simulink model "Simulink_TEP"  (R2024a)
settings: Solver=FixedStepAuto  StartTime=0.0  StopTime=5  FixedStep=1/3600  RelTol=1e-3
model workspace (MAT data in the model file):
  AD : Simulink.Parameter (value not decoded)
  AG : Simulink.Parameter (value not decoded)
  AH : Simulink.Parameter (value not decoded)
  AV : Simulink.Parameter (value not decoded)
  AVP : Simulink.Parameter (value not decoded)
  BCHL : Simulink.Parameter (value not decoded)
  BCHV : Simulink.Parameter (value not decoded)
  BD : Simulink.Parameter (value not decoded)
  BG : Simulink.Parameter (value not decoded)
  BH : Simulink.Parameter (value not decoded)
  BVP : Simulink.Parameter (value not decoded)
  CD : Simulink.Parameter (value not decoded)
  CG : Simulink.Parameter (value not decoded)
  CH : Simulink.Parameter (value not decoded)
  CVP : Simulink.Parameter (value not decoded)
  XMW : Simulink.Parameter (value not decoded)
symbols that are objects in the model workspace (value not decoded): AD, AG, AH, AV, AVP, BD, BG, BH, BVP, CD, CG, CH, CVP, XMW
undefined symbols (not defined in the file or in its folder): magnitude, SETPT, XMEAS, XMV
libraries: mylib x165, dspindex x17
(part 9 of 10)

== system Simulink_TEP/Subsystem/Braatz/ 9/CONTROL 16 ==
  XMEAS(18) : Inport
  SETPT(16) : Inport  Port=2
  Constant1 : Constant  Value=GAIN16
  Constant2 : Constant  Value=TAUI16
  Constant3 : Constant  Value=HIGH16
  Constant5 : Constant  Value=SI16
  Constant6 : Constant  Value=HIGH9
  PI Control Setpoint : mylib/Braatz Control/PI Control Setpoint  SystemSampleTime=-1  VariantActivationTime=update diagram  AllowFlexibleInterface=on  Latency=0  AutoFrameSizeCalculation=off
  Sampling interval : mylib/Braatz Control/Sampling interval  SystemSampleTime=-1  VariantActivationTime=update diagram  AllowFlexibleInterface=on  Latency=0  AutoFrameSizeCalculation=off
  Unit Delay : UnitDelay  InitialCondition=SETPT9  SampleTime=-1  HasFrameUpgradeWarning=on
  Unit Delay1 : UnitDelay  SampleTime=-1  HasFrameUpgradeWarning=on
  SETPT(9) : Outport  VectorParamsAs1DForOutWhenUnconnected=off
  wires:
  Sampling interval/1 -> PI Control Setpoint/Action
  SETPT(16)/1 -> PI Control Setpoint/1
  XMEAS(18)/1 -> PI Control Setpoint/2
  PI Control Setpoint/1 -> SETPT(9)/1, Unit Delay/1
  Constant2/1 -> PI Control Setpoint/8
  Constant5/1 -> PI Control Setpoint/7, Sampling interval/1
  Constant1/1 -> PI Control Setpoint/6
  Constant3/1 -> PI Control Setpoint/3
  Unit Delay/1 -> PI Control Setpoint/4
  Constant6/1 -> PI Control Setpoint/5
  PI Control Setpoint/2 -> Unit Delay1/1
  Unit Delay1/1 -> PI Control Setpoint/9

== system Simulink_TEP/Subsystem/Braatz/ 9/CONTROL 20 ==
  XMEAS(38) : Inport
  Constant : Constant  Value=SETPT20
  Constant1 : Constant  Value=GAIN20
  Constant2 : Constant  Value=TAUI20
  Constant3 : Constant  Value=HIGH20
  Constant5 : Constant  Value=SI20
  Constant6 : Constant  Value=HIGH16
  PI Control Setpoint : mylib/Braatz Control/PI Control Setpoint  SystemSampleTime=-1  VariantActivationTime=update diagram  AllowFlexibleInterface=on  Latency=0  AutoFrameSizeCalculation=off
  Sampling interval : mylib/Braatz Control/Sampling interval  SystemSampleTime=-1  VariantActivationTime=update diagram  AllowFlexibleInterface=on  Latency=0  AutoFrameSizeCalculation=off
  Unit Delay : UnitDelay  InitialCondition=SETPT16  SampleTime=-1  HasFrameUpgradeWarning=on
  Unit Delay1 : UnitDelay  SampleTime=-1  HasFrameUpgradeWarning=on
  SETPT(16) : Outport  VectorParamsAs1DForOutWhenUnconnected=off
  wires:
  Sampling interval/1 -> PI Control Setpoint/Action
  Constant/1 -> PI Control Setpoint/1
  XMEAS(38)/1 -> PI Control Setpoint/2
  PI Control Setpoint/1 -> SETPT(16)/1, Unit Delay/1
  Constant2/1 -> PI Control Setpoint/8
  Constant5/1 -> PI Control Setpoint/7, Sampling interval/1
  Constant1/1 -> PI Control Setpoint/6
  Constant3/1 -> PI Control Setpoint/3
  Unit Delay/1 -> PI Control Setpoint/4
  Constant6/1 -> PI Control Setpoint/5
  PI Control Setpoint/2 -> Unit Delay1/1
  Unit Delay1/1 -> PI Control Setpoint/9

== system Simulink_TEP/Subsystem/Braatz/ 9/CONTROL 9 ==
  XMEAS(19) : Inport
  SETPT(9) : Inport  Port=2
  Constant1 : Constant  Value=GAIN9
  Constant2 : Constant  Value=HIGH9
  Constant3 : Constant  Value=SI9
  P Control : mylib/Braatz Control/P Control  SystemSampleTime=-1  VariantActivationTime=update diagram  AllowFlexibleInterface=on  Latency=0  AutoFrameSizeCalculation=off
  Sampling interval : mylib/Braatz Control/Sampling interval  SystemSampleTime=-1  VariantActivationTime=update diagram  AllowFlexibleInterface=on  Latency=0  AutoFrameSizeCalculation=off
  Unit Delay : UnitDelay  InitialCondition=XMV9_0  SampleTime=-1  HasFrameUpgradeWarning=on
  Unit Delay1 : UnitDelay  SampleTime=-1  HasFrameUpgradeWarning=on
  XMV(9) : Outport  VectorParamsAs1DForOutWhenUnconnected=off
  wires:
  Constant2/1 -> P Control/5
  Constant1/1 -> P Control/3
  SETPT(9)/1 -> P Control/1
  Unit Delay/1 -> P Control/2
  XMEAS(19)/1 -> P Control/4
  P Control/1 -> XMV(9)/1, Unit Delay/1
  Sampling interval/1 -> P Control/Action
  Constant3/1 -> Sampling interval/1
  P Control/2 -> Unit Delay1/1
  Unit Delay1/1 -> P Control/6

== system Simulink_TEP/Disturbances/Subsystem1/Subsystem2/If Action Subsystem/Subsystem ==
  Bus Creator : BusCreator  Inputs=5
  HSPAN(2) : Constant  Value=0.7
  HZERO(2) : Constant
  SPSPAN(2) : Constant  Value=0
  SSPAN(2) : Constant  Value=0.003
  SZERO(2) : Constant  Value=0.005
  Out1 : Outport  VectorParamsAs1DForOutWhenUnconnected=off
  wires:
  SSPAN(2)/1 -> Bus Creator/3  "SSPAN"
  HSPAN(2)/1 -> Bus Creator/1  "HSPAN"
  Bus Creator/1 -> Out1/1
  SPSPAN(2)/1 -> Bus Creator/5  "SPSPAN"
  HZERO(2)/1 -> Bus Creator/2  "HZERO"
  SZERO(2)/1 -> Bus Creator/4  "SZERO"

== system Simulink_TEP/Disturbances/Subsystem1/Subsystem2/If Action Subsystem1/Subsystem1 ==
  BDIST(2) : Constant  Value=0
  Bus Creator : BusCreator  Inputs=6
  CDIST(2) : Constant  Value=0
  DDIST(2) : Constant  Value=0
  SZERO(2) : Constant  Value=0.005
  TENXT(2) : Constant  Value=0.1
  TLAST(2) : Constant  Value=0
  DIST : Outport  VectorParamsAs1DForOutWhenUnconnected=off
  wires:
  Bus Creator/1 -> DIST/1
  TENXT(2)/1 -> Bus Creator/5  "TNEXT"
  SZERO(2)/1 -> Bus Creator/1  "ADIST"
  TLAST(2)/1 -> Bus Creator/6  "TLAST"
  DDIST(2)/1 -> Bus Creator/4  "DDIST"
  BDIST(2)/1 -> Bus Creator/2  "BDIST"
  CDIST(2)/1 -> Bus Creator/3  "CDIST"

== system Simulink_TEP/Disturbances/Subsystem10/Subsystem3/If Action Subsystem/Subsystem2 ==
  Bus Creator : BusCreator  Inputs=5
  HSPAN(10) : Constant  Value=1.5
  HZERO(10) : Constant  Value=2
  SPSPAN(10) : Constant  Value=0
  SSPAN(10) : Constant  Value=0
  SZERO(10) : Constant  Value=0
  Out1 : Outport  VectorParamsAs1DForOutWhenUnconnected=off
  wires:
  SSPAN(10)/1 -> Bus Creator/3  "SSPAN"
  HSPAN(10)/1 -> Bus Creator/1  "HSPAN"
  Bus Creator/1 -> Out1/1
  SPSPAN(10)/1 -> Bus Creator/5  "SPSPAN"
  HZERO(10)/1 -> Bus Creator/2  "HZERO"
  SZERO(10)/1 -> Bus Creator/4  "SZERO"

== system Simulink_TEP/Disturbances/Subsystem10/Subsystem3/If Action Subsystem1/Subsystem1 ==
  BDIST(10) : Constant  Value=0
  Bus Creator : BusCreator  Inputs=6
  CDIST(10) : Constant  Value=0
  DDIST(10) : Constant  Value=0
  SZERO(10) : Constant  Value=0
  TENXT(10) : Constant  Value=0.1
  TLAST(10) : Constant  Value=0
  DIST : Outport  VectorParamsAs1DForOutWhenUnconnected=off
  wires:
  Bus Creator/1 -> DIST/1
  TENXT(10)/1 -> Bus Creator/5  "TNEXT"
  SZERO(10)/1 -> Bus Creator/1  "ADIST"
  TLAST(10)/1 -> Bus Creator/6  "TLAST"
  DDIST(10)/1 -> Bus Creator/4  "DDIST"
  BDIST(10)/1 -> Bus Creator/2  "BDIST"
  CDIST(10)/1 -> Bus Creator/3  "CDIST"

== system Simulink_TEP/Disturbances/Subsystem11/Subsystem3/If Action Subsystem/Subsystem2 ==
  Bus Creator : BusCreator  Inputs=5
  HSPAN(11) : Constant  Value=2
  HZERO(11) : Constant  Value=3
  SPSPAN(11) : Constant  Value=0
  SSPAN(11) : Constant  Value=0
  SZERO(11) : Constant  Value=0
  Out1 : Outport  VectorParamsAs1DForOutWhenUnconnected=off
  wires:
  SSPAN(11)/1 -> Bus Creator/3  "SSPAN"
  HSPAN(11)/1 -> Bus Creator/1  "HSPAN"
  Bus Creator/1 -> Out1/1
  SPSPAN(11)/1 -> Bus Creator/5  "SPSPAN"
  HZERO(11)/1 -> Bus Creator/2  "HZERO"
  SZERO(11)/1 -> Bus Creator/4  "SZERO"

== system Simulink_TEP/Disturbances/Subsystem11/Subsystem3/If Action Subsystem1/Subsystem1 ==
  BDIST(11) : Constant  Value=0
  Bus Creator : BusCreator  Inputs=6
  CDIST(11) : Constant  Value=0
  DDIST(11) : Constant  Value=0
  SZERO(11) : Constant  Value=0
  TENXT(11) : Constant  Value=0.1
  TLAST(11) : Constant  Value=0
  DIST : Outport  VectorParamsAs1DForOutWhenUnconnected=off
  wires:
  Bus Creator/1 -> DIST/1
  TENXT(11)/1 -> Bus Creator/5  "TNEXT"
  SZERO(11)/1 -> Bus Creator/1  "ADIST"
  TLAST(11)/1 -> Bus Creator/6  "TLAST"
  DDIST(11)/1 -> Bus Creator/4  "DDIST"
  BDIST(11)/1 -> Bus Creator/2  "BDIST"
  CDIST(11)/1 -> Bus Creator/3  "CDIST"

== system Simulink_TEP/Disturbances/Subsystem12/Subsystem3/If Action Subsystem/Subsystem2 ==
  Bus Creator : BusCreator  Inputs=5
  HSPAN(12) : Constant  Value=1.5
  HZERO(12) : Constant  Value=2
  SPSPAN(12) : Constant  Value=0
  SSPAN(12) : Constant  Value=0
  SZERO(12) : Constant  Value=0
  Out1 : Outport  VectorParamsAs1DForOutWhenUnconnected=off
  wires:
  SSPAN(12)/1 -> Bus Creator/3  "SSPAN"
  HSPAN(12)/1 -> Bus Creator/1  "HSPAN"
  Bus Creator/1 -> Out1/1
  SPSPAN(12)/1 -> Bus Creator/5  "SPSPAN"
  HZERO(12)/1 -> Bus Creator/2  "HZERO"
  SZERO(12)/1 -> Bus Creator/4  "SZERO"

== system Simulink_TEP/Disturbances/Subsystem12/Subsystem3/If Action Subsystem1/Subsystem1 ==
  BDIST(12) : Constant  Value=0
  Bus Creator : BusCreator  Inputs=6
  CDIST(12) : Constant  Value=0
  DDIST(12) : Constant  Value=0
  SZERO(12) : Constant  Value=0
  TENXT(12) : Constant  Value=0.1
  TLAST(12) : Constant  Value=0
  DIST : Outport  VectorParamsAs1DForOutWhenUnconnected=off
  wires:
  Bus Creator/1 -> DIST/1
  TENXT(12)/1 -> Bus Creator/5  "TNEXT"
  SZERO(12)/1 -> Bus Creator/1  "ADIST"
  TLAST(12)/1 -> Bus Creator/6  "TLAST"
  DDIST(12)/1 -> Bus Creator/4  "DDIST"
  BDIST(12)/1 -> Bus Creator/2  "BDIST"
  CDIST(12)/1 -> Bus Creator/3  "CDIST"

== system Simulink_TEP/Disturbances/Subsystem2/Subsystem/If Action Subsystem/Subsystem ==
  Bus Creator : BusCreator  Inputs=5
  HSPAN(1) : Constant  Value=0.2
  HZERO(1) : Constant  Value=0.5
  SPSPAN(1) : Constant  Value=0
  SSPAN(1) : Constant  Value=0.03
  SZERO(1) : Constant  Value=0.485
  Out1 : Outport  VectorParamsAs1DForOutWhenUnconnected=off
  wires:
  SSPAN(1)/1 -> Bus Creator/3  "SSPAN"
  HSPAN(1)/1 -> Bus Creator/1  "HSPAN"
  Bus Creator/1 -> Out1/1
  SPSPAN(1)/1 -> Bus Creator/5  "SPSPAN"
  HZERO(1)/1 -> Bus Creator/2  "HZERO"
  SZERO(1)/1 -> Bus Creator/4  "SZERO"

== system Simulink_TEP/Disturbances/Subsystem2/Subsystem/If Action Subsystem1/Subsystem1 ==
  BDIST(1) : Constant  Value=0
  Bus Creator : BusCreator  Inputs=6
  CDIST(1) : Constant  Value=0
  DDIST(1) : Constant  Value=0
  SZERO(1) : Constant  Value=0.485
  TENXT(1) : Constant  Value=0.1
  TLAST(1) : Constant  Value=0
  DIST : Outport  VectorParamsAs1DForOutWhenUnconnected=off
  wires:
  Bus Creator/1 -> DIST/1
  TENXT(1)/1 -> Bus Creator/5  "TNEXT"
  SZERO(1)/1 -> Bus Creator/1  "ADIST"
  TLAST(1)/1 -> Bus Creator/6  "TLAST"
  DDIST(1)/1 -> Bus Creator/4  "DDIST"
  BDIST(1)/1 -> Bus Creator/2  "BDIST"
  CDIST(1)/1 -> Bus Creator/3  "CDIST"

== system Simulink_TEP/Disturbances/Subsystem3/Subsystem2/If Action Subsystem/Subsystem ==
  Bus Creator : BusCreator  Inputs=5
  HSPAN(3) : Constant  Value=0.25
  HZERO(3) : Constant  Value=0.5
  SPSPAN(3) : Constant  Value=0
  SSPAN(3) : Constant  Value=10
  SZERO(3) : Constant  Value=45
  Out1 : Outport  VectorParamsAs1DForOutWhenUnconnected=off
  wires:
  SSPAN(3)/1 -> Bus Creator/3  "SSPAN"
  HSPAN(3)/1 -> Bus Creator/1  "HSPAN"
  Bus Creator/1 -> Out1/1
  SPSPAN(3)/1 -> Bus Creator/5  "SPSPAN"
  HZERO(3)/1 -> Bus Creator/2  "HZERO"
  SZERO(3)/1 -> Bus Creator/4  "SZERO"

== system Simulink_TEP/Disturbances/Subsystem3/Subsystem2/If Action Subsystem1/Subsystem1 ==
  BDIST(3) : Constant  Value=0
  Bus Creator : BusCreator  Inputs=6
  CDIST(3) : Constant  Value=0
  DDIST(3) : Constant  Value=0
  SZERO(3) : Constant  Value=45
  TENXT(3) : Constant  Value=0.1
  TLAST(3) : Constant  Value=0
  DIST : Outport  VectorParamsAs1DForOutWhenUnconnected=off
  wires:
  Bus Creator/1 -> DIST/1
  TENXT(3)/1 -> Bus Creator/5  "TNEXT"
  SZERO(3)/1 -> Bus Creator/1  "ADIST"
  TLAST(3)/1 -> Bus Creator/6  "TLAST"
  DDIST(3)/1 -> Bus Creator/4  "DDIST"
  BDIST(3)/1 -> Bus Creator/2  "BDIST"
  CDIST(3)/1 -> Bus Creator/3  "CDIST"

== system Simulink_TEP/Disturbances/Subsystem4/Subsystem2/If Action Subsystem/Subsystem ==
  Bus Creator : BusCreator  Inputs=5
  HSPAN(4) : Constant  Value=0.7
  HZERO(4) : Constant
  SPSPAN(4) : Constant  Value=0
  SSPAN(4) : Constant  Value=10
  SZERO(4) : Constant  Value=45
  Out1 : Outport  VectorParamsAs1DForOutWhenUnconnected=off
  wires:
  SSPAN(4)/1 -> Bus Creator/3  "SSPAN"
  HSPAN(4)/1 -> Bus Creator/1  "HSPAN"
  Bus Creator/1 -> Out1/1
  SPSPAN(4)/1 -> Bus Creator/5  "SPSPAN"
  HZERO(4)/1 -> Bus Creator/2  "HZERO"
  SZERO(4)/1 -> Bus Creator/4  "SZERO"

== system Simulink_TEP/Disturbances/Subsystem4/Subsystem2/If Action Subsystem1/Subsystem1 ==
  BDIST(4) : Constant  Value=0
  Bus Creator : BusCreator  Inputs=6
  CDIST(4) : Constant  Value=0
  DDIST(4) : Constant  Value=0
  SZERO(4) : Constant  Value=45
  TENXT(4) : Constant  Value=0.1
  TLAST(4) : Constant  Value=0
  DIST : Outport  VectorParamsAs1DForOutWhenUnconnected=off
  wires:
  Bus Creator/1 -> DIST/1
  TENXT(4)/1 -> Bus Creator/5  "TNEXT"
  SZERO(4)/1 -> Bus Creator/1  "ADIST"
  TLAST(4)/1 -> Bus Creator/6  "TLAST"
  DDIST(4)/1 -> Bus Creator/4  "DDIST"
  BDIST(4)/1 -> Bus Creator/2  "BDIST"
  CDIST(4)/1 -> Bus Creator/3  "CDIST"

== system Simulink_TEP/Disturbances/Subsystem5/Subsystem2/If Action Subsystem/Subsystem ==
  Bus Creator : BusCreator  Inputs=5
  HSPAN(5) : Constant  Value=0.15
  HZERO(5) : Constant  Value=0.25
  SPSPAN(5) : Constant  Value=0
  SSPAN(5) : Constant  Value=10
  SZERO(5) : Constant  Value=35
  Out1 : Outport  VectorParamsAs1DForOutWhenUnconnected=off
  wires:
  SSPAN(5)/1 -> Bus Creator/3  "SSPAN"
  HSPAN(5)/1 -> Bus Creator/1  "HSPAN"
  Bus Creator/1 -> Out1/1
  SPSPAN(5)/1 -> Bus Creator/5  "SPSPAN"
  HZERO(5)/1 -> Bus Creator/2  "HZERO"
  SZERO(5)/1 -> Bus Creator/4  "SZERO"

== system Simulink_TEP/Disturbances/Subsystem5/Subsystem2/If Action Subsystem1/Subsystem1 ==
  BDIST(5) : Constant  Value=0
  Bus Creator : BusCreator  Inputs=6
  CDIST(5) : Constant  Value=0
  DDIST(5) : Constant  Value=0
  SZERO(5) : Constant  Value=35
  TENXT(5) : Constant  Value=0.1
  TLAST(5) : Constant  Value=0
  DIST : Outport  VectorParamsAs1DForOutWhenUnconnected=off
  wires:
  Bus Creator/1 -> DIST/1
  TENXT(5)/1 -> Bus Creator/5  "TNEXT"
  SZERO(5)/1 -> Bus Creator/1  "ADIST"
  TLAST(5)/1 -> Bus Creator/6  "TLAST"
  DDIST(5)/1 -> Bus Creator/4  "DDIST"
  BDIST(5)/1 -> Bus Creator/2  "BDIST"
  CDIST(5)/1 -> Bus Creator/3  "CDIST"

== system Simulink_TEP/Disturbances/Subsystem6/Subsystem2/If Action Subsystem/Subsystem ==
  Bus Creator : BusCreator  Inputs=5
  HSPAN(6) : Constant  Value=0.15
  HZERO(6) : Constant  Value=0.25
  SPSPAN(6) : Constant  Value=0
  SSPAN(6) : Constant  Value=10
  SZERO(6) : Constant  Value=40
  Out1 : Outport  VectorParamsAs1DForOutWhenUnconnected=off
  wires:
  SSPAN(6)/1 -> Bus Creator/3  "SSPAN"
  HSPAN(6)/1 -> Bus Creator/1  "HSPAN"
  Bus Creator/1 -> Out1/1
  SPSPAN(6)/1 -> Bus Creator/5  "SPSPAN"
  HZERO(6)/1 -> Bus Creator/2  "HZERO"
  SZERO(6)/1 -> Bus Creator/4  "SZERO"

== system Simulink_TEP/Disturbances/Subsystem6/Subsystem2/If Action Subsystem1/Subsystem1 ==
  BDIST(6) : Constant  Value=0
  Bus Creator : BusCreator  Inputs=6
  CDIST(6) : Constant  Value=0
  DDIST(6) : Constant  Value=0
  SZERO(6) : Constant  Value=40
  TENXT(6) : Constant  Value=0.1
  TLAST(6) : Constant  Value=0
  DIST : Outport  VectorParamsAs1DForOutWhenUnconnected=off
  wires:
  Bus Creator/1 -> DIST/1
  TENXT(6)/1 -> Bus Creator/5  "TNEXT"
  SZERO(6)/1 -> Bus Creator/1  "ADIST"
  TLAST(6)/1 -> Bus Creator/6  "TLAST"
  DDIST(6)/1 -> Bus Creator/4  "DDIST"
  BDIST(6)/1 -> Bus Creator/2  "BDIST"
  CDIST(6)/1 -> Bus Creator/3  "CDIST"

== system Simulink_TEP/Disturbances/Subsystem7/Subsystem2/If Action Subsystem/Subsystem ==
  Bus Creator : BusCreator  Inputs=5
  HSPAN(7) : Constant
  HZERO(7) : Constant  Value=2
  SPSPAN(7) : Constant  Value=0
  SSPAN(7) : Constant  Value=0.25
  SZERO(7) : Constant
  Out1 : Outport  VectorParamsAs1DForOutWhenUnconnected=off
  wires:
  SSPAN(7)/1 -> Bus Creator/3  "SSPAN"
  HSPAN(7)/1 -> Bus Creator/1  "HSPAN"
  Bus Creator/1 -> Out1/1
  SPSPAN(7)/1 -> Bus Creator/5  "SPSPAN"
  HZERO(7)/1 -> Bus Creator/2  "HZERO"
  SZERO(7)/1 -> Bus Creator/4  "SZERO"

== system Simulink_TEP/Disturbances/Subsystem7/Subsystem2/If Action Subsystem1/Subsystem1 ==
  BDIST(7) : Constant  Value=0
  Bus Creator : BusCreator  Inputs=6
  CDIST(7) : Constant  Value=0
  DDIST(7) : Constant  Value=0
  SZERO(7) : Constant
  TENXT(7) : Constant  Value=0.1
  TLAST(7) : Constant  Value=0
  DIST : Outport  VectorParamsAs1DForOutWhenUnconnected=off
  wires:
  Bus Creator/1 -> DIST/1
  TENXT(7)/1 -> Bus Creator/5  "TNEXT"
  SZERO(7)/1 -> Bus Creator/1  "ADIST"
  TLAST(7)/1 -> Bus Creator/6  "TLAST"
  DDIST(7)/1 -> Bus Creator/4  "DDIST"
  BDIST(7)/1 -> Bus Creator/2  "BDIST"
  CDIST(7)/1 -> Bus Creator/3  "CDIST"

== system Simulink_TEP/Disturbances/Subsystem8/Subsystem2/If Action Subsystem/Subsystem ==
  Bus Creator : BusCreator  Inputs=5
  HSPAN(8) : Constant
  HZERO(8) : Constant  Value=2
  SPSPAN(8) : Constant  Value=0
  SSPAN(8) : Constant  Value=0.25
  SZERO(8) : Constant
  Out1 : Outport  VectorParamsAs1DForOutWhenUnconnected=off
  wires:
  SSPAN(8)/1 -> Bus Creator/3  "SSPAN"
  HSPAN(8)/1 -> Bus Creator/1  "HSPAN"
  Bus Creator/1 -> Out1/1
  SPSPAN(8)/1 -> Bus Creator/5  "SPSPAN"
  HZERO(8)/1 -> Bus Creator/2  "HZERO"
  SZERO(8)/1 -> Bus Creator/4  "SZERO"

== system Simulink_TEP/Disturbances/Subsystem8/Subsystem2/If Action Subsystem1/Subsystem1 ==
  BDIST(8) : Constant  Value=0
  Bus Creator : BusCreator  Inputs=6
  CDIST(8) : Constant  Value=0
  DDIST(8) : Constant  Value=0
  SZERO(8) : Constant
  TENXT(8) : Constant  Value=0.1
  TLAST(8) : Constant  Value=0
  DIST : Outport  VectorParamsAs1DForOutWhenUnconnected=off
  wires:
  Bus Creator/1 -> DIST/1
  TENXT(8)/1 -> Bus Creator/5  "TNEXT"
  SZERO(8)/1 -> Bus Creator/1  "ADIST"
  TLAST(8)/1 -> Bus Creator/6  "TLAST"
  DDIST(8)/1 -> Bus Creator/4  "DDIST"
  BDIST(8)/1 -> Bus Creator/2  "BDIST"
  CDIST(8)/1 -> Bus Creator/3  "CDIST"

== system Simulink_TEP/Disturbances/Subsystem9/Subsystem2/If Action Subsystem/Subsystem ==
  Bus Creator : BusCreator  Inputs=5
  HSPAN(9) : Constant  Value=0.4
  HZERO(9) : Constant  Value=0.5
  SPSPAN(9) : Constant  Value=0
  SSPAN(9) : Constant  Value=0.25
  SZERO(9) : Constant  Value=0
  Out1 : Outport  VectorParamsAs1DForOutWhenUnconnected=off
  wires:
  SSPAN(9)/1 -> Bus Creator/3  "SSPAN"
  HSPAN(9)/1 -> Bus Creator/1  "HSPAN"
  Bus Creator/1 -> Out1/1
  SPSPAN(9)/1 -> Bus Creator/5  "SPSPAN"
  HZERO(9)/1 -> Bus Creator/2  "HZERO"
  SZERO(9)/1 -> Bus Creator/4  "SZERO"

== system Simulink_TEP/Disturbances/Subsystem9/Subsystem2/If Action Subsystem1/Subsystem1 ==
  BDIST(9) : Constant  Value=0
  Bus Creator : BusCreator  Inputs=6
  CDIST(9) : Constant  Value=0
  DDIST(9) : Constant  Value=0
  SZERO(9) : Constant  Value=0
  TENXT(9) : Constant  Value=0.1
  TLAST(9) : Constant  Value=0
  DIST : Outport  VectorParamsAs1DForOutWhenUnconnected=off
  wires:
  Bus Creator/1 -> DIST/1
  TENXT(9)/1 -> Bus Creator/5  "TNEXT"
  SZERO(9)/1 -> Bus Creator/1  "ADIST"
  TLAST(9)/1 -> Bus Creator/6  "TLAST"
  DDIST(9)/1 -> Bus Creator/4  "DDIST"
  BDIST(9)/1 -> Bus Creator/2  "BDIST"
  CDIST(9)/1 -> Bus Creator/3  "CDIST"

== system Simulink_TEP/Random number generator/Disturbances I=1-9/TESUB7(1)/Subsystem/If Action Subsystem ==
  In1 : Inport
  Action Port : ActionPort  ActionPortLabel=if(u1 == 0)
  Out1 : Outport  VectorParamsAs1DForOutWhenUnconnected=off
  wires:
  In1/1 -> Out1/1

== system Simulink_TEP/Random number generator/Disturbances I=1-9/TESUB7(1)/Subsystem/If Action Subsystem1 ==
  In1 : Inport
  Action Port : ActionPort  ActionPortLabel=else
  Out1 : Outport  VectorParamsAs1DForOutWhenUnconnected=off
  wires:
  In1/1 -> Out1/1

== system Simulink_TEP/Random number generator/Disturbances I=1-9/TESUB7(2)/Subsystem/If Action Subsystem ==
  In1 : Inport
  Action Port : ActionPort  ActionPortLabel=if(u1 == 0)
  Out1 : Outport  VectorParamsAs1DForOutWhenUnconnected=off
  wires:
  In1/1 -> Out1/1

== system Simulink_TEP/Random number generator/Disturbances I=1-9/TESUB7(2)/Subsystem/If Action Subsystem1 ==
  In1 : Inport
  Action Port : ActionPort  ActionPortLabel=else
  Out1 : Outport  VectorParamsAs1DForOutWhenUnconnected=off
  wires:
  In1/1 -> Out1/1

== system Simulink_TEP/Random number generator/Disturbances I=1-9/TESUB7(3)/Subsystem/If Action Subsystem ==
  In1 : Inport
  Action Port : ActionPort  ActionPortLabel=if(u1 == 0)
  Out1 : Outport  VectorParamsAs1DForOutWhenUnconnected=off
  wires:
  In1/1 -> Out1/1

== system Simulink_TEP/Random number generator/Disturbances I=1-9/TESUB7(3)/Subsystem/If Action Subsystem1 ==
  In1 : Inport
  Action Port : ActionPort  ActionPortLabel=else
  Out1 : Outport  VectorParamsAs1DForOutWhenUnconnected=off
  wires:
  In1/1 -> Out1/1

== system Simulink_TEP/Random number generator/Disturbances I=1-9/TESUB7(4)/Subsystem/If Action Subsystem ==
  In1 : Inport
  Action Port : ActionPort  ActionPortLabel=if(u1 == 0)
  Out1 : Outport  VectorParamsAs1DForOutWhenUnconnected=off
  wires:
  In1/1 -> Out1/1

== system Simulink_TEP/Random number generator/Disturbances I=1-9/TESUB7(4)/Subsystem/If Action Subsystem1 ==
  In1 : Inport
  Action Port : ActionPort  ActionPortLabel=else
  Out1 : Outport  VectorParamsAs1DForOutWhenUnconnected=off
  wires:
  In1/1 -> Out1/1

== system Simulink_TEP/Random number generator/Disturbances I=1-9/TESUB7(5)/Subsystem/If Action Subsystem ==
  In1 : Inport
  Action Port : ActionPort  ActionPortLabel=if(u1 == 0)
  Out1 : Outport  VectorParamsAs1DForOutWhenUnconnected=off
  wires:
  In1/1 -> Out1/1

== system Simulink_TEP/Random number generator/Disturbances I=1-9/TESUB7(5)/Subsystem/If Action Subsystem1 ==
  In1 : Inport
  Action Port : ActionPort  ActionPortLabel=else
  Out1 : Outport  VectorParamsAs1DForOutWhenUnconnected=off
  wires:
  In1/1 -> Out1/1

== system Simulink_TEP/Random number generator/Disturbances I=1-9/TESUB7(6)/Subsystem/If Action Subsystem ==
  In1 : Inport
  Action Port : ActionPort  ActionPortLabel=if(u1 == 0)
  Out1 : Outport  VectorParamsAs1DForOutWhenUnconnected=off
  wires:
  In1/1 -> Out1/1

== system Simulink_TEP/Random number generator/Disturbances I=1-9/TESUB7(6)/Subsystem/If Action Subsystem1 ==
  In1 : Inport
  Action Port : ActionPort  ActionPortLabel=else
  Out1 : Outport  VectorParamsAs1DForOutWhenUnconnected=off
  wires:
  In1/1 -> Out1/1

== system Simulink_TEP/Random number generator/Disturbances I=1-9/TESUB7(7)/Subsystem/If Action Subsystem ==
  In1 : Inport
  Action Port : ActionPort  ActionPortLabel=if(u1 == 0)
  Out1 : Outport  VectorParamsAs1DForOutWhenUnconnected=off
  wires:
  In1/1 -> Out1/1

== system Simulink_TEP/Random number generator/Disturbances I=1-9/TESUB7(7)/Subsystem/If Action Subsystem1 ==
  In1 : Inport
  Action Port : ActionPort  ActionPortLabel=else
  Out1 : Outport  VectorParamsAs1DForOutWhenUnconnected=off
  wires:
  In1/1 -> Out1/1

== system Simulink_TEP/Random number generator/Disturbances I=1-9/TESUB7(8)/Subsystem/If Action Subsystem ==
  In1 : Inport
  Action Port : ActionPort  ActionPortLabel=if(u1 == 0)
  Out1 : Outport  VectorParamsAs1DForOutWhenUnconnected=off
  wires:
  In1/1 -> Out1/1

== system Simulink_TEP/Random number generator/Disturbances I=1-9/TESUB7(8)/Subsystem/If Action Subsystem1 ==
  In1 : Inport
  Action Port : ActionPort  ActionPortLabel=else
  Out1 : Outport  VectorParamsAs1DForOutWhenUnconnected=off
  wires:
  In1/1 -> Out1/1

== system Simulink_TEP/Random number generator/Disturbances I=1-9/TESUB7(9)/Subsystem/If Action Subsystem ==
  In1 : Inport
  Action Port : ActionPort  ActionPortLabel=if(u1 == 0)
  Out1 : Outport  VectorParamsAs1DForOutWhenUnconnected=off
  wires:
  In1/1 -> Out1/1

== system Simulink_TEP/Random number generator/Disturbances I=1-9/TESUB7(9)/Subsystem/If Action Subsystem1 ==
  In1 : Inport
  Action Port : ActionPort  ActionPortLabel=else
  Out1 : Outport  VectorParamsAs1DForOutWhenUnconnected=off
  wires:
  In1/1 -> Out1/1

== system Simulink_TEP/Random number generator/Disturbances I=10-12/TESUB7(10)/Subsystem/If Action Subsystem ==
  In1 : Inport
  Action Port : ActionPort  ActionPortLabel=if(u1 == 0)
  Out1 : Outport  VectorParamsAs1DForOutWhenUnconnected=off
  wires:
  In1/1 -> Out1/1

== system Simulink_TEP/Random number generator/Disturbances I=10-12/TESUB7(10)/Subsystem/If Action Subsystem1 ==
  In1 : Inport
  Action Port : ActionPort  ActionPortLabel=else
  Out1 : Outport  VectorParamsAs1DForOutWhenUnconnected=off
  wires:
  In1/1 -> Out1/1

== system Simulink_TEP/Random number generator/Disturbances I=10-12/TESUB7(11)/Subsystem/If Action Subsystem ==
  In1 : Inport
  Action Port : ActionPort  ActionPortLabel=if(u1 == 0)
  Out1 : Outport  VectorParamsAs1DForOutWhenUnconnected=off
  wires:
  In1/1 -> Out1/1

== system Simulink_TEP/Random number generator/Disturbances I=10-12/TESUB7(11)/Subsystem/If Action Subsystem1 ==
  In1 : Inport
  Action Port : ActionPort  ActionPortLabel=else
  Out1 : Outport  VectorParamsAs1DForOutWhenUnconnected=off
  wires:
  In1/1 -> Out1/1

== system Simulink_TEP/Random number generator/Disturbances I=10-12/TESUB7(12)/Subsystem/If Action Subsystem ==
  In1 : Inport
  Action Port : ActionPort  ActionPortLabel=if(u1 == 0)
  Out1 : Outport  VectorParamsAs1DForOutWhenUnconnected=off
  wires:
  In1/1 -> Out1/1

== system Simulink_TEP/Random number generator/Disturbances I=10-12/TESUB7(12)/Subsystem/If Action Subsystem1 ==
  In1 : Inport
  Action Port : ActionPort  ActionPortLabel=else
  Out1 : Outport  VectorParamsAs1DForOutWhenUnconnected=off
  wires:
  In1/1 -> Out1/1

== system Simulink_TEP/Random number generator/Process Measurements XMEAS(I) I=1-22/If Action Subsystem3/Subsystem/Subsystem ==
  G : Inport
  TESUB6 XMNS(1) : Subsystem
  TESUB6 XMNS(2) : Subsystem
  TESUB6 XMNS(3) : Subsystem
  TESUB6 XMNS(4) : Subsystem
  TESUB6 XMNS(5) : Subsystem
  XMNS(1) : Outport  VectorParamsAs1DForOutWhenUnconnected=off
  XMNS(2) : Outport  Port=2  VectorParamsAs1DForOutWhenUnconnected=off
  XMNS(3) : Outport  Port=3  VectorParamsAs1DForOutWhenUnconnected=off
  XMNS(4) : Outport  Port=4  VectorParamsAs1DForOutWhenUnconnected=off
  XMNS(5) : Outport  Port=5  VectorParamsAs1DForOutWhenUnconnected=off
  G_NEW : Outport  Port=6  VectorParamsAs1DForOutWhenUnconnected=off
  wires:
  TESUB6 XMNS(2)/2(G_NEW) -> TESUB6 XMNS(3)/1(G)
  G/1 -> TESUB6 XMNS(1)/1(G)
  TESUB6 XMNS(1)/2(G_NEW) -> TESUB6 XMNS(2)/1(G)
  TESUB6 XMNS(3)/2(G_NEW) -> TESUB6 XMNS(4)/1(G)
  TESUB6 XMNS(4)/1(XMNS) -> XMNS(4)/1  "XMNS(4)"
  TESUB6 XMNS(5)/1(XMNS) -> XMNS(5)/1  "XMNS(5)"
  TESUB6 XMNS(5)/2(G_NEW) -> G_NEW/1
  TESUB6 XMNS(4)/2(G_NEW) -> TESUB6 XMNS(5)/1(G)
  TESUB6 XMNS(3)/1(XMNS) -> XMNS(3)/1  "XMNS(3)"
  TESUB6 XMNS(1)/1(XMNS) -> XMNS(1)/1  "XMNS(1)"
  TESUB6 XMNS(2)/1(XMNS) -> XMNS(2)/1  "XMNS(2)"

== system Simulink_TEP/Random number generator/Process Measurements XMEAS(I) I=1-22/If Action Subsystem3/Subsystem/Subsystem1 ==
  G : Inport
  TESUB6 XMNS(10) : Subsystem
  TESUB6 XMNS(6) : Subsystem
  TESUB6 XMNS(7) : Subsystem
  TESUB6 XMNS(8) : Subsystem
  TESUB6 XMNS(9) : Subsystem
  XMNS(6) : Outport  VectorParamsAs1DForOutWhenUnconnected=off
  XMNS(7) : Outport  Port=2  VectorParamsAs1DForOutWhenUnconnected=off
  XMNS(8) : Outport  Port=3  VectorParamsAs1DForOutWhenUnconnected=off
  XMNS(9) : Outport  Port=4  VectorParamsAs1DForOutWhenUnconnected=off
  XMNS(10) : Outport  Port=5  VectorParamsAs1DForOutWhenUnconnected=off
  G_NEW : Outport  Port=6  VectorParamsAs1DForOutWhenUnconnected=off
  wires:
  TESUB6 XMNS(7)/2(G_NEW) -> TESUB6 XMNS(8)/1(G)
  G/1 -> TESUB6 XMNS(6)/1(G)
  TESUB6 XMNS(6)/2(G_NEW) -> TESUB6 XMNS(7)/1(G)
  TESUB6 XMNS(8)/2(G_NEW) -> TESUB6 XMNS(9)/1(G)
  TESUB6 XMNS(9)/1(XMNS) -> XMNS(9)/1  "XMNS(9)"
  TESUB6 XMNS(10)/1(XMNS) -> XMNS(10)/1  "XMNS(10)"
  TESUB6 XMNS(10)/2(G_NEW) -> G_NEW/1
  TESUB6 XMNS(9)/2(G_NEW) -> TESUB6 XMNS(10)/1(G)
  TESUB6 XMNS(8)/1(XMNS) -> XMNS(8)/1  "XMNS(8)"
  TESUB6 XMNS(6)/1(XMNS) -> XMNS(6)/1  "XMNS(6)"
  TESUB6 XMNS(7)/1(XMNS) -> XMNS(7)/1  "XMNS(7)"

== system Simulink_TEP/Random number generator/Process Measurements XMEAS(I) I=1-22/If Action Subsystem3/Subsystem/Subsystem2 ==
  G : Inport
  TESUB6 XMNS(11) : Subsystem
  TESUB6 XMNS(12) : Subsystem
  TESUB6 XMNS(13) : Subsystem
  TESUB6 XMNS(14) : Subsystem
  TESUB6 XMNS(15) : Subsystem
  XMNS(11) : Outport  VectorParamsAs1DForOutWhenUnconnected=off
  XMNS(12) : Outport  Port=2  VectorParamsAs1DForOutWhenUnconnected=off
  XMNS(13) : Outport  Port=3  VectorParamsAs1DForOutWhenUnconnected=off
  XMNS(14) : Outport  Port=4  VectorParamsAs1DForOutWhenUnconnected=off
  XMNS(15) : Outport  Port=5  VectorParamsAs1DForOutWhenUnconnected=off
  G_NEW : Outport  Port=6  VectorParamsAs1DForOutWhenUnconnected=off
  wires:
  TESUB6 XMNS(12)/2(G_NEW) -> TESUB6 XMNS(13)/1(G)
  G/1 -> TESUB6 XMNS(11)/1(G)
  TESUB6 XMNS(11)/2(G_NEW) -> TESUB6 XMNS(12)/1(G)
  TESUB6 XMNS(13)/2(G_NEW) -> TESUB6 XMNS(14)/1(G)
  TESUB6 XMNS(14)/1(XMNS) -> XMNS(14)/1  "XMNS(14)"
  TESUB6 XMNS(15)/1(XMNS) -> XMNS(15)/1  "XMNS(15)"
  TESUB6 XMNS(15)/2(G_NEW) -> G_NEW/1
  TESUB6 XMNS(14)/2(G_NEW) -> TESUB6 XMNS(15)/1(G)
  TESUB6 XMNS(13)/1(XMNS) -> XMNS(13)/1  "XMNS(13)"
  TESUB6 XMNS(11)/1(XMNS) -> XMNS(11)/1  "XMNS(11)"
  TESUB6 XMNS(12)/1(XMNS) -> XMNS(12)/1  "XMNS(12)"

== system Simulink_TEP/Random number generator/Process Measurements XMEAS(I) I=1-22/If Action Subsystem3/Subsystem/Subsystem3 ==
  G : Inport
  TESUB6 XMNS(16) : Subsystem
  TESUB6 XMNS(17) : Subsystem
  TESUB6 XMNS(18) : Subsystem
  TESUB6 XMNS(19) : Subsystem
  TESUB6 XMNS(20) : Subsystem
  TESUB6 XMNS(21) : Subsystem
  TESUB6 XMNS(22) : Subsystem
  XMNS(16) : Outport  VectorParamsAs1DForOutWhenUnconnected=off
  XMNS(17) : Outport  Port=2  VectorParamsAs1DForOutWhenUnconnected=off
  XMNS(18) : Outport  Port=3  VectorParamsAs1DForOutWhenUnconnected=off
  XMNS(19) : Outport  Port=4  VectorParamsAs1DForOutWhenUnconnected=off
  XMNS(20) : Outport  Port=5  VectorParamsAs1DForOutWhenUnconnected=off
  XMNS(21) : Outport  Port=6  VectorParamsAs1DForOutWhenUnconnected=off
  XMNS(22) : Outport  Port=7  VectorParamsAs1DForOutWhenUnconnected=off
  G_NEW : Outport  Port=8  VectorParamsAs1DForOutWhenUnconnected=off
  wires:
  TESUB6 XMNS(17)/2(G_NEW) -> TESUB6 XMNS(18)/1(G)
  G/1 -> TESUB6 XMNS(16)/1(G)
  TESUB6 XMNS(16)/2(G_NEW) -> TESUB6 XMNS(17)/1(G)
  TESUB6 XMNS(18)/2(G_NEW) -> TESUB6 XMNS(19)/1(G)
  TESUB6 XMNS(19)/1(XMNS) -> XMNS(19)/1  "XMNS(19)"
  TESUB6 XMNS(20)/1(XMNS) -> XMNS(20)/1  "XMNS(20)"
  TESUB6 XMNS(18)/1(XMNS) -> XMNS(18)/1  "XMNS(18)"
  TESUB6 XMNS(16)/1(XMNS) -> XMNS(16)/1  "XMNS(16)"
  TESUB6 XMNS(17)/1(XMNS) -> XMNS(17)/1  "XMNS(17)"
  TESUB6 XMNS(21)/1(XMNS) -> XMNS(21)/1  "XMNS(21)"
  TESUB6 XMNS(22)/1(XMNS) -> XMNS(22)/1  "XMNS(22)"
  TESUB6 XMNS(22)/2(G_NEW) -> G_NEW/1
  TESUB6 XMNS(20)/2(G_NEW) -> TESUB6 XMNS(21)/1(G)
  TESUB6 XMNS(21)/2(G_NEW) -> TESUB6 XMNS(22)/1(G)
  TESUB6 XMNS(19)/2(G_NEW) -> TESUB6 XMNS(20)/1(G)

== system Simulink_TEP/Random number generator/Process Measurements XMEAS(I) I=23-36/If Action Subsystem3/Subsystem/Subsystem ==
  G : Inport
  TESUB6 XMNS(23) : Subsystem
  TESUB6 XMNS(24) : Subsystem
  TESUB6 XMNS(25) : Subsystem
  TESUB6 XMNS(26) : Subsystem
  TESUB6 XMNS(27) : Subsystem
  XMNS(23) : Outport  VectorParamsAs1DForOutWhenUnconnected=off
  XMNS(24) : Outport  Port=2  VectorParamsAs1DForOutWhenUnconnected=off
  XMNS(25) : Outport  Port=3  VectorParamsAs1DForOutWhenUnconnected=off
  XMNS(26) : Outport  Port=4  VectorParamsAs1DForOutWhenUnconnected=off
  XMNS(27) : Outport  Port=5  VectorParamsAs1DForOutWhenUnconnected=off
  G_NEW : Outport  Port=6  VectorParamsAs1DForOutWhenUnconnected=off
  wires:
  TESUB6 XMNS(24)/2(G_NEW) -> TESUB6 XMNS(25)/1(G)
  G/1 -> TESUB6 XMNS(23)/1(G)
  TESUB6 XMNS(23)/2(G_NEW) -> TESUB6 XMNS(24)/1(G)
  TESUB6 XMNS(25)/2(G_NEW) -> TESUB6 XMNS(26)/1(G)
  TESUB6 XMNS(26)/1(XMNS) -> XMNS(26)/1  "XMNS(26)"
  TESUB6 XMNS(27)/1(XMNS) -> XMNS(27)/1  "XMNS(27)"
  TESUB6 XMNS(27)/2(G_NEW) -> G_NEW/1
  TESUB6 XMNS(26)/2(G_NEW) -> TESUB6 XMNS(27)/1(G)
  TESUB6 XMNS(25)/1(XMNS) -> XMNS(25)/1  "XMNS(25)"
  TESUB6 XMNS(23)/1(XMNS) -> XMNS(23)/1  "XMNS(23)"
  TESUB6 XMNS(24)/1(XMNS) -> XMNS(24)/1  "XMNS(24)"

== system Simulink_TEP/Random number generator/Process Measurements XMEAS(I) I=23-36/If Action Subsystem3/Subsystem/Subsystem1 ==
  G : Inport
  TESUB6 XMNS(28) : Subsystem
  TESUB6 XMNS(29) : Subsystem
  TESUB6 XMNS(30) : Subsystem
  TESUB6 XMNS(31) : Subsystem
  TESUB6 XMNS(32) : Subsystem
  XMNS(28) : Outport  VectorParamsAs1DForOutWhenUnconnected=off
  XMNS(29) : Outport  Port=2  VectorParamsAs1DForOutWhenUnconnected=off
  XMNS(30) : Outport  Port=3  VectorParamsAs1DForOutWhenUnconnected=off
  XMNS(31) : Outport  Port=4  VectorParamsAs1DForOutWhenUnconnected=off
  XMNS(32) : Outport  Port=5  VectorParamsAs1DForOutWhenUnconnected=off
  G_NEW : Outport  Port=6  VectorParamsAs1DForOutWhenUnconnected=off
  wires:
  TESUB6 XMNS(29)/2(G_NEW) -> TESUB6 XMNS(30)/1(G)
  G/1 -> TESUB6 XMNS(28)/1(G)
  TESUB6 XMNS(28)/2(G_NEW) -> TESUB6 XMNS(29)/1(G)
  TESUB6 XMNS(30)/2(G_NEW) -> TESUB6 XMNS(31)/1(G)
  TESUB6 XMNS(31)/1(XMNS) -> XMNS(31)/1  "XMNS(31)"
  TESUB6 XMNS(32)/1(XMNS) -> XMNS(32)/1  "XMNS(32)"
  TESUB6 XMNS(32)/2(G_NEW) -> G_NEW/1
  TESUB6 XMNS(31)/2(G_NEW) -> TESUB6 XMNS(32)/1(G)
  TESUB6 XMNS(30)/1(XMNS) -> XMNS(30)/1  "XMNS(30)"
  TESUB6 XMNS(28)/1(XMNS) -> XMNS(28)/1  "XMNS(28)"
  TESUB6 XMNS(29)/1(XMNS) -> XMNS(29)/1  "XMNS(29)"

== system Simulink_TEP/Random number generator/Process Measurements XMEAS(I) I=23-36/If Action Subsystem3/Subsystem/Subsystem2 ==
  G : Inport
  TESUB6 XMNS(33) : Subsystem
  TESUB6 XMNS(34) : Subsystem
  TESUB6 XMNS(35) : Subsystem
  TESUB6 XMNS(36) : Subsystem
  XMNS(33) : Outport  VectorParamsAs1DForOutWhenUnconnected=off
  XMNS(34) : Outport  Port=2  VectorParamsAs1DForOutWhenUnconnected=off
  XMNS(35) : Outport  Port=3  VectorParamsAs1DForOutWhenUnconnected=off
  XMNS(36) : Outport  Port=4  VectorParamsAs1DForOutWhenUnconnected=off
  G_NEW : Outport  Port=5  VectorParamsAs1DForOutWhenUnconnected=off
  wires:
  TESUB6 XMNS(34)/2(G_NEW) -> TESUB6 XMNS(35)/1(G)
  G/1 -> TESUB6 XMNS(33)/1(G)
  TESUB6 XMNS(33)/2(G_NEW) -> TESUB6 XMNS(34)/1(G)
  TESUB6 XMNS(35)/2(G_NEW) -> TESUB6 XMNS(36)/1(G)
  TESUB6 XMNS(36)/1(XMNS) -> XMNS(36)/1  "XMNS(36)"
  TESUB6 XMNS(36)/2(G_NEW) -> G_NEW/1
  TESUB6 XMNS(35)/1(XMNS) -> XMNS(35)/1  "XMNS(35)"
  TESUB6 XMNS(33)/1(XMNS) -> XMNS(33)/1  "XMNS(33)"
  TESUB6 XMNS(34)/1(XMNS) -> XMNS(34)/1  "XMNS(34)"

== system Simulink_TEP/Random number generator/Process Measurements XMEAS(I) I=37-41/If Action Subsystem3/Subsystem/Subsystem ==
  G : Inport
  TESUB6 XMNS(37) : Subsystem
  TESUB6 XMNS(38) : Subsystem
  TESUB6 XMNS(39) : Subsystem
  TESUB6 XMNS(40) : Subsystem
  TESUB6 XMNS(41) : Subsystem
  XMNS(37) : Outport  VectorParamsAs1DForOutWhenUnconnected=off
  XMNS(38) : Outport  Port=2  VectorParamsAs1DForOutWhenUnconnected=off
  XMNS(39) : Outport  Port=3  VectorParamsAs1DForOutWhenUnconnected=off
  XMNS(40) : Outport  Port=4  VectorParamsAs1DForOutWhenUnconnected=off
  XMNS(41) : Outport  Port=5  VectorParamsAs1DForOutWhenUnconnected=off
  G_NEW : Outport  Port=6  VectorParamsAs1DForOutWhenUnconnected=off
  wires:
  TESUB6 XMNS(38)/2(G_NEW) -> TESUB6 XMNS(39)/1(G)
  G/1 -> TESUB6 XMNS(37)/1(G)
  TESUB6 XMNS(37)/2(G_NEW) -> TESUB6 XMNS(38)/1(G)
  TESUB6 XMNS(39)/2(G_NEW) -> TESUB6 XMNS(40)/1(G)
  TESUB6 XMNS(40)/1(XMNS) -> XMNS(40)/1  "XMNS(40)"
  TESUB6 XMNS(41)/1(XMNS) -> XMNS(41)/1  "XMNS(41)"
  TESUB6 XMNS(41)/2(G_NEW) -> G_NEW/1
  TESUB6 XMNS(40)/2(G_NEW) -> TESUB6 XMNS(41)/1(G)
  TESUB6 XMNS(39)/1(XMNS) -> XMNS(39)/1  "XMNS(39)"
  TESUB6 XMNS(37)/1(XMNS) -> XMNS(37)/1  "XMNS(37)"
  TESUB6 XMNS(38)/1(XMNS) -> XMNS(38)/1  "XMNS(38)"

== system Simulink_TEP/Reactor/Reaction Rates/Reaction rates lb-mol//h/Reaction rate of reaction 1 lb-mol//ft3·h/If Action Subsystem ==
  In1 : Inport
  Action Port : ActionPort  ActionPortLabel=if( u1>0 & u2>0 )
  Out1 : Outport  VectorParamsAs1DForOutWhenUnconnected=off
  wires:
  In1/1 -> Out1/1

== system Simulink_TEP/Reactor/Reaction Rates/Reaction rates lb-mol//h/Reaction rate of reaction 1 lb-mol//ft3·h/If Action Subsystem2 ==
  In1 : Inport
  Action Port : ActionPort  ActionPortLabel=else
  Out1 : Outport  VectorParamsAs1DForOutWhenUnconnected=off
  wires:
  In1/1 -> Out1/1

== system Simulink_TEP/Reactor/Reaction Rates/Reaction rates lb-mol//h/Reaction rate of reaction 1 lb-mol//ft3·h/RR(1) Reaction rate of 1st reaction lb-mol//ft3·h  ==
  PPR : Inport
  TKR : Inport  Port=2
  "   " : Constant  Value=1.1544
  "    " : Constant  Value=0.3735
  Abs : Abs  SaturateOnIntegerOverflow=off
  Abs1 : Abs  SaturateOnIntegerOverflow=off
  Activation energy cal/mol : Constant  Value=40000
  Bus Selector : BusSelector  OutputSignals=PPR(1),PPR(3),PPR(4)
  Bus Selector1 : BusSelector  OutputSignals=TESUB8(7)
  Divide : Product  Inputs=*//
  Divide1 : Product  Inputs=4
  Math Function1 : Math  SignedPower=on
  Preexponential factor lb-mol/ft3·h·mmHg : Constant  Value=31.5859536
  Product : Product
  R1F : Math  Operator=pow  SignedPower=on
  R2F : Math  Operator=pow  SignedPower=on
  Subtract : Sum  Inputs=+-
  Universal gas constant cal/mol·K : Constant  Value=1.987
  RR(1) : Outport  VectorParamsAs1DForOutWhenUnconnected=off
  wires:
  "    "/1 -> R2F/2
  Divide/1 -> Subtract/2
  Universal gas constant cal/mol·K/1 -> Divide/2
  "   "/1 -> R1F/2
  Preexponential factor lb-mol/ft3·h·mmHg/1 -> Subtract/1
  Activation energy cal/mol/1 -> Divide/1
  TKR/1 -> Divide/3
  Subtract/1 -> Math Function1/1
  Divide1/1 -> RR(1)/1
  Bus Selector/2 -> Abs1/1  "<PPR(3)>"
  Abs/1 -> R1F/1
  Abs1/1 -> R2F/1
  PPR/1 -> Bus Selector/1
  Bus Selector/1 -> Abs/1  "<PPR(1)>"
  R1F/1 -> Divide1/2
  R2F/1 -> Divide1/3
  Bus Selector/3 -> Divide1/4  "<PPR(4)>"
  [TESUB8] -> Bus Selector1/1
  Math Function1/1 -> Product/1
  Bus Selector1/1 -> Product/2  "<TESUB8(7)>"
  Product/1 -> Divide1/1

== system Simulink_TEP/Reactor/Reaction Rates/Reaction rates lb-mol//h/Reaction rate of reaction 2 lb-mol//ft3·h/If Action Subsystem ==
  In1 : Inport
  Action Port : ActionPort  ActionPortLabel=if( u1>0 & u2>0)
  Out1 : Outport  VectorParamsAs1DForOutWhenUnconnected=off
  wires:
  In1/1 -> Out1/1

== system Simulink_TEP/Reactor/Reaction Rates/Reaction rates lb-mol//h/Reaction rate of reaction 2 lb-mol//ft3·h/If Action Subsystem2 ==
  In1 : Inport
  Action Port : ActionPort  ActionPortLabel=else
  Out1 : Outport  VectorParamsAs1DForOutWhenUnconnected=off
  wires:
  In1/1 -> Out1/1

== system Simulink_TEP/Reactor/Reaction Rates/Reaction rates lb-mol//h/Reaction rate of reaction 2 lb-mol//ft3·h/RR(2) Reaction rate of 2nd reaction lb-mol//ft3·h  ==
  PPR : Inport
  TKR : Inport  Port=2
  "   " : Constant  Value=1.1544
  "    " : Constant  Value=0.3735
  Abs : Abs  SaturateOnIntegerOverflow=off
  Abs1 : Abs  SaturateOnIntegerOverflow=off
  Activation energy cal/mol : Constant  Value=20000
  Bus Selector : BusSelector  OutputSignals=PPR(1),PPR(3),PPR(5)
  Bus Selector1 : BusSelector  OutputSignals=TESUB8(8)
  Divide : Product  Inputs=*//
  Divide1 : Product  Inputs=4
  Math Function2 : Math  SignedPower=on
  Preexponential factor lb-mol/ft3·h·mmHg : Constant  Value=3.00094014
  Product : Product
  R1F : Math  Operator=pow  SignedPower=on
  R2F : Math  Operator=pow  SignedPower=on
  Subtract : Sum  Inputs=+-
  Universal gas constant cal/mol·K : Constant  Value=1.987
  RR(2) : Outport  VectorParamsAs1DForOutWhenUnconnected=off
  wires:
  "    "/1 -> R2F/2
  Divide/1 -> Subtract/2
  Universal gas constant cal/mol·K/1 -> Divide/2
  "   "/1 -> R1F/2
  Preexponential factor lb-mol/ft3·h·mmHg/1 -> Subtract/1
  Activation energy cal/mol/1 -> Divide/1
  TKR/1 -> Divide/3
  Subtract/1 -> Math Function2/1
  Divide1/1 -> RR(2)/1
  Bus Selector/2 -> Abs1/1  "<PPR(3)>"
  Abs/1 -> R1F/1
  Abs1/1 -> R2F/1
  PPR/1 -> Bus Selector/1
  Bus Selector/1 -> Abs/1  "<PPR(1)>"
  R1F/1 -> Divide1/2
  R2F/1 -> Divide1/3
  Bus Selector/3 -> Divide1/4  "<PPR(5)>"
  [TESUB8] -> Bus Selector1/1
  Product/1 -> Divide1/1
  Math Function2/1 -> Product/1
  Bus Selector1/1 -> Product/2  "<TESUB8(8)>"

== system Simulink_TEP/Reactor/Reactor Heat exchanger/Reactor Heat exchanger/Subsystem/If Action Subsystem ==
  In1 : Inport
  Action Port : ActionPort  ActionPortLabel=if(u1 > 50)
  Out1 : Outport  VectorParamsAs1DForOutWhenUnconnected=off
  wires:
  In1/1 -> Out1/1

== system Simulink_TEP/Reactor/Reactor Heat exchanger/Reactor Heat exchanger/Subsystem/If Action Subsystem1 ==
  In1 : Inport
  Action Port : ActionPort  ActionPortLabel=elseif(u1 < 10)
  Out1 : Outport  VectorParamsAs1DForOutWhenUnconnected=off
  wires:
  In1/1 -> Out1/1

== system Simulink_TEP/Reactor/Reactor Heat exchanger/Reactor Heat exchanger/Subsystem/If Action Subsystem2 ==
  In1 : Inport
  Action Port : ActionPort  ActionPortLabel=else
  Out1 : Outport  VectorParamsAs1DForOutWhenUnconnected=off
  wires:
  In1/1 -> Out1/1

== system Simulink_TEP/Reactor/Reactor Heat exchanger/Reactor Heat exchanger/Subsystem1/TCWR ==
  Add : Sum
  Bus Selector : BusSelector  OutputSignals=TESUB8(5)
  Bus Selector1 : BusSelector  OutputSignals=IDV(4)
  Constant : Constant  Value=5
  Product1 : Product
  TCWR : Outport  VectorParamsAs1DForOutWhenUnconnected=off
  wires:
  Constant/1 -> Product1/2
  Bus Selector/1 -> Add/1  "<TESUB8(5)>"
  Bus Selector1/1 -> Product1/1  "<IDV(4)>"
  [TESUB8] -> Bus Selector/1
  Product1/1 -> Add/2
  [IDV] -> Bus Selector1/1
  Add/1 -> TCWR/1

== system Simulink_TEP/Separator/Stream 9/Subsystem/Pressure drop/If Action Subsystem ==
  In1 : Inport
  Action Port : ActionPort  ActionPortLabel=if(u1 < 0)
  Out1 : Outport  VectorParamsAs1DForOutWhenUnconnected=off
  wires:
  In1/1 -> Out1/1

== system Simulink_TEP/Separator/Stream 9/Subsystem/Pressure drop/If Action Subsystem1 ==
  In1 : Inport
  Action Port : ActionPort  ActionPortLabel=else
  Out1 : Outport  VectorParamsAs1DForOutWhenUnconnected=off
  wires:
  In1/1 -> Out1/1

== system Simulink_TEP/Subsystem/Braatz/ 10/CONTROL 6/P Control ==
  SETPT : Inport
  XMV_OLD : Inport  Port=2
  GAIN : Inport  Port=3
  XMEAS : Inport  Port=4
  High Limit : Inport  Port=5
  Action Port : ActionPort  ActionPortLabel=if(u1 == 0)
  Add1 : Sum
  ERR : Subsystem
  Pressure limits : Subsystem
      mask Display: color('Blue'),disp('Pressure limits'),
  Subsystem : Subsystem
  XMV_NEW : Outport  VectorParamsAs1DForOutWhenUnconnected=off
  wires:
  High Limit/1 -> ERR/2(High Limit)
  GAIN/1 -> Subsystem/2(GAIN)
  Pressure limits/1(XMV(6)) -> XMV_NEW/1
  SETPT/1 -> ERR/1(SETPT)
  XMV_OLD/1 -> Add1/2
  Add1/1 -> Pressure limits/1("XMV(6) ")  "XMV"
  Subsystem/1(DXMV) -> Add1/1  "DXMV"
  ERR/1(ERR) -> Subsystem/1(ERR)
  XMEAS/1 -> ERR/3(XMEAS), Pressure limits/2(XMEAS)

== system Simulink_TEP/Random number generator/Process Measurements XMEAS(I) I=1-22/If Action Subsystem3/Subsystem/Subsystem/TESUB6 XMNS(1) ==
  G : Inport
  Process Noise I=1-12 G New : mylib/Process Noise I=1-12 G New  SystemSampleTime=-1  VariantActivationTime=update diagram  AllowFlexibleInterface=on  Latency=0  AutoFrameSizeCalculation=off
  XNS(1) : Constant  Value=0.0012
  XMNS : Outport  VectorParamsAs1DForOutWhenUnconnected=off
  G_NEW : Outport  Port=2  VectorParamsAs1DForOutWhenUnconnected=off
  wires:
  XNS(1)/1 -> Process Noise I=1-12 G New/1
  Process Noise I=1-12 G New/1 -> XMNS/1
  G/1 -> Process Noise I=1-12 G New/2
  Process Noise I=1-12 G New/2 -> G_NEW/1

== system Simulink_TEP/Random number generator/Process Measurements XMEAS(I) I=1-22/If Action Subsystem3/Subsystem/Subsystem/TESUB6 XMNS(2) ==
  G : Inport
  Process Noise I=1-12 G New : mylib/Process Noise I=1-12 G New  SystemSampleTime=-1  VariantActivationTime=update diagram  AllowFlexibleInterface=on  Latency=0  AutoFrameSizeCalculation=off
  XNS(2) : Constant  Value=18.000
  XMNS : Outport  VectorParamsAs1DForOutWhenUnconnected=off
  G_NEW : Outport  Port=2  VectorParamsAs1DForOutWhenUnconnected=off
  wires:
  XNS(2)/1 -> Process Noise I=1-12 G New/1
  Process Noise I=1-12 G New/1 -> XMNS/1
  G/1 -> Process Noise I=1-12 G New/2
  Process Noise I=1-12 G New/2 -> G_NEW/1

== system Simulink_TEP/Random number generator/Process Measurements XMEAS(I) I=1-22/If Action Subsystem3/Subsystem/Subsystem/TESUB6 XMNS(3) ==
  G : Inport
  Process Noise I=1-12 G New : mylib/Process Noise I=1-12 G New  SystemSampleTime=-1  VariantActivationTime=update diagram  AllowFlexibleInterface=on  Latency=0  AutoFrameSizeCalculation=off
  XNS(3) : Constant  Value=22.000
  XMNS : Outport  VectorParamsAs1DForOutWhenUnconnected=off
  G_NEW : Outport  Port=2  VectorParamsAs1DForOutWhenUnconnected=off
  wires:
  XNS(3)/1 -> Process Noise I=1-12 G New/1
  Process Noise I=1-12 G New/1 -> XMNS/1
  G/1 -> Process Noise I=1-12 G New/2
  Process Noise I=1-12 G New/2 -> G_NEW/1

== system Simulink_TEP/Random number generator/Process Measurements XMEAS(I) I=1-22/If Action Subsystem3/Subsystem/Subsystem/TESUB6 XMNS(4) ==
  G : Inport
  Process Noise I=1-12 G New : mylib/Process Noise I=1-12 G New  SystemSampleTime=-1  VariantActivationTime=update diagram  AllowFlexibleInterface=on  Latency=0  AutoFrameSizeCalculation=off
  XNS(4) : Constant  Value=0.0500
  XMNS : Outport  VectorParamsAs1DForOutWhenUnconnected=off
  G_NEW : Outport  Port=2  VectorParamsAs1DForOutWhenUnconnected=off
  wires:
  XNS(4)/1 -> Process Noise I=1-12 G New/1
  Process Noise I=1-12 G New/1 -> XMNS/1
  G/1 -> Process Noise I=1-12 G New/2
  Process Noise I=1-12 G New/2 -> G_NEW/1

== system Simulink_TEP/Random number generator/Process Measurements XMEAS(I) I=1-22/If Action Subsystem3/Subsystem/Subsystem/TESUB6 XMNS(5) ==
  G : Inport
  Process Noise I=1-12 G New : mylib/Process Noise I=1-12 G New  SystemSampleTime=-1  VariantActivationTime=update diagram  AllowFlexibleInterface=on  Latency=0  AutoFrameSizeCalculation=off
  XNS(5) : Constant  Value=0.2000
  XMNS : Outport  VectorParamsAs1DForOutWhenUnconnected=off
  G_NEW : Outport  Port=2  VectorParamsAs1DForOutWhenUnconnected=off
  wires:
  XNS(5)/1 -> Process Noise I=1-12 G New/1
  Process Noise I=1-12 G New/1 -> XMNS/1
  G/1 -> Process Noise I=1-12 G New/2
  Process Noise I=1-12 G New/2 -> G_NEW/1

== system Simulink_TEP/Random number generator/Process Measurements XMEAS(I) I=1-22/If Action Subsystem3/Subsystem/Subsystem1/TESUB6 XMNS(10) ==
  G : Inport
  Process Noise I=1-12 G New : mylib/Process Noise I=1-12 G New  SystemSampleTime=-1  VariantActivationTime=update diagram  AllowFlexibleInterface=on  Latency=0  AutoFrameSizeCalculation=off
  XNS(10) : Constant  Value=0.0017
  XMNS : Outport  VectorParamsAs1DForOutWhenUnconnected=off
  G_NEW : Outport  Port=2  VectorParamsAs1DForOutWhenUnconnected=off
  wires:
  XNS(10)/1 -> Process Noise I=1-12 G New/1
  Process Noise I=1-12 G New/1 -> XMNS/1
  G/1 -> Process Noise I=1-12 G New/2
  Process Noise I=1-12 G New/2 -> G_NEW/1

== system Simulink_TEP/Random number generator/Process Measurements XMEAS(I) I=1-22/If Action Subsystem3/Subsystem/Subsystem1/TESUB6 XMNS(6) ==
  G : Inport
  Process Noise I=1-12 G New : mylib/Process Noise I=1-12 G New  SystemSampleTime=-1  VariantActivationTime=update diagram  AllowFlexibleInterface=on  Latency=0  AutoFrameSizeCalculation=off
  XNS(6) : Constant  Value=0.2100
  XMNS : Outport  VectorParamsAs1DForOutWhenUnconnected=off
  G_NEW : Outport  Port=2  VectorParamsAs1DForOutWhenUnconnected=off
  wires:
  XNS(6)/1 -> Process Noise I=1-12 G New/1
  Process Noise I=1-12 G New/1 -> XMNS/1
  G/1 -> Process Noise I=1-12 G New/2
  Process Noise I=1-12 G New/2 -> G_NEW/1

== system Simulink_TEP/Random number generator/Process Measurements XMEAS(I) I=1-22/If Action Subsystem3/Subsystem/Subsystem1/TESUB6 XMNS(7) ==
  G : Inport
  Process Noise I=1-12 G New : mylib/Process Noise I=1-12 G New  SystemSampleTime=-1  VariantActivationTime=update diagram  AllowFlexibleInterface=on  Latency=0  AutoFrameSizeCalculation=off
  XNS(7) : Constant  Value=0.3000
  XMNS : Outport  VectorParamsAs1DForOutWhenUnconnected=off
  G_NEW : Outport  Port=2  VectorParamsAs1DForOutWhenUnconnected=off
  wires:
  XNS(7)/1 -> Process Noise I=1-12 G New/1
  Process Noise I=1-12 G New/1 -> XMNS/1
  G/1 -> Process Noise I=1-12 G New/2
  Process Noise I=1-12 G New/2 -> G_NEW/1

== system Simulink_TEP/Random number generator/Process Measurements XMEAS(I) I=1-22/If Action Subsystem3/Subsystem/Subsystem1/TESUB6 XMNS(8) ==
  G : Inport
  Display1 : Display
  Process Noise I=1-12 G New : mylib/Process Noise I=1-12 G New  SystemSampleTime=-1  VariantActivationTime=update diagram  AllowFlexibleInterface=on  Latency=0  AutoFrameSizeCalculation=off
  XNS(8) : Constant  Value=0.5000
  XMNS : Outport  VectorParamsAs1DForOutWhenUnconnected=off
  G_NEW : Outport  Port=2  VectorParamsAs1DForOutWhenUnconnected=off
  wires:
  XNS(8)/1 -> Process Noise I=1-12 G New/1
  Process Noise I=1-12 G New/1 -> XMNS/1
  G/1 -> Display1/1, Process Noise I=1-12 G New/2
  Process Noise I=1-12 G New/2 -> G_NEW/1
